simulink library "EngU2Cnt_lib"  (Simulink 7.2)
settings: Solver=ode45  SolverMode=SingleTasking  StartTime=0.0  StopTime=10.0  RelTol=1e-3
undefined symbols (not defined in the file or in its folder): RefGainBias_Vec
libraries: simulink x1
settings Model: Creator=cbuttril  LastModifiedBy=amurch

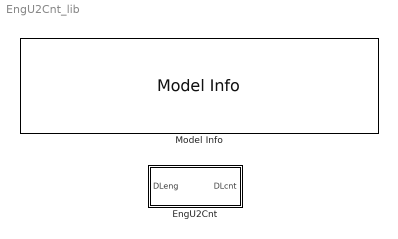
== system EngU2Cnt_lib ==
  EngU2Cnt : Subsystem
  Model Info : simulink/Model-Wide Utilities/Model Info  SystemSampleTime=-1  InitialBlockCM=None  BlockCM=None  Frame=on  DisplayStringWithTags=|  HorizontalTextAlignment=Center  LeftAlignmentValue=0.5  SourceBlockDiagram=EngU2Cnt_lib  TagMaxNumber=20
      | Developed using Matlab Release 2007a
      | 
      | SVN:%<ModelVersion>
      | Last modifed by %<LastModifiedBy> on %<LastModificationDate>

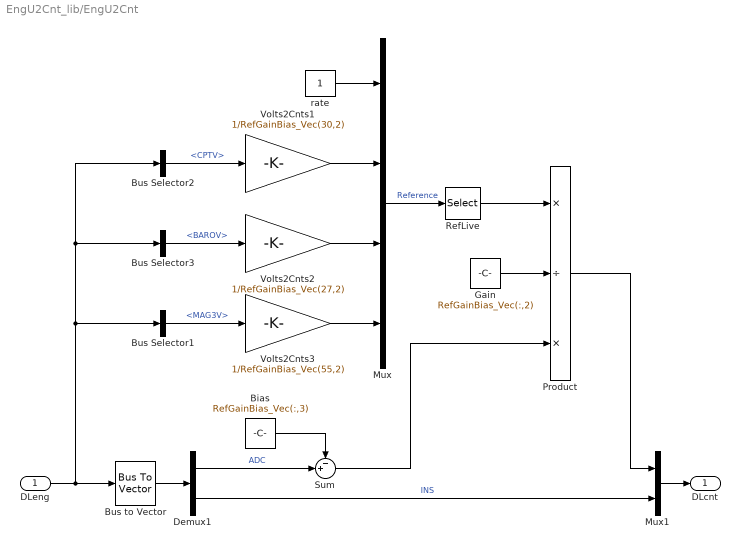
== system EngU2Cnt_lib/EngU2Cnt ==
  DLeng : Inport  OutDataType=sfix(16)  OutScaling=2^0
  Bias : Constant  Value=RefGainBias_Vec(:,3)  OutDataType=sfix(16)  OutScaling=2^0
  Bus Selector1 : BusSelector  OutputSignals=ADC.MAG3V
  Bus Selector2 : BusSelector  OutputSignals=ADC.CPTV
  Bus Selector3 : BusSelector  OutputSignals=ADC.BAROV
  Bus to Vector : BusToVector
  Demux1 : Demux  Outputs=[62 99]
  Gain : Constant  Value=RefGainBias_Vec(:,2)  OutDataType=sfix(16)  OutScaling=2^0
  Mux : Mux
  Mux1 : Mux  Inputs=2
  Product : Product  Inputs=*/*  OutDataType=sfix(16)  OutScaling=2^0  RndMeth=Zero
  RefLive : Selector  IndexMode=Zero-based  InputPortWidth=4  IndexOptions=Index vector (dialog)  Indices=RefGainBias_Vec(:,1)  OutputSizes=1
  Sum : Sum  Inputs=-+|  OutDataType=sfix(16)  OutScaling=2^0
  Volts2Cnts1 : Gain  Gain=1/RefGainBias_Vec(30,2)  ParameterDataType=sfix(16)  ParameterScaling=2^0  OutDataType=sfix(16)  OutScaling=2^0
  Volts2Cnts2 : Gain  Gain=1/RefGainBias_Vec(27,2)  ParameterDataType=sfix(16)  ParameterScaling=2^0  OutDataType=sfix(16)  OutScaling=2^0
  Volts2Cnts3 : Gain  Gain=1/RefGainBias_Vec(55,2)  ParameterDataType=sfix(16)  ParameterScaling=2^0  OutDataType=sfix(16)  OutScaling=2^0
  rate : Constant  OutDataType=sfix(16)  OutScaling=2^0
  DLcnt : Outport  OutDataType=sfix(16)  OutScaling=2^0
  wires:
  Bus Selector3/1 -> Volts2Cnts2/1  "<BAROV>"
  Mux1/1 -> DLcnt/1
  Demux1/2 -> Mux1/2  "INS"
  Demux1/1 -> Sum/2  "ADC"
  Bias/1 -> Sum/1
  Bus to Vector/1 -> Demux1/1
  DLeng/1 -> Bus to Vector/1, Bus Selector1/1, Bus Selector2/1, Bus Selector3/1
  Mux/1 -> RefLive/1  "Reference"
  rate/1 -> Mux/1
  Bus Selector2/1 -> Volts2Cnts1/1  "<CPTV>"
  Bus Selector1/1 -> Volts2Cnts3/1  "<MAG3V>"
  Product/1 -> Mux1/1
  RefLive/1 -> Product/1
  Gain/1 -> Product/2
  Sum/1 -> Product/3
  Volts2Cnts1/1 -> Mux/2
  Volts2Cnts2/1 -> Mux/3
  Volts2Cnts3/1 -> Mux/4
